simulink model "racecar_shiftlight"  (R2023b)
settings: Solver=FixedStepAuto  StartTime=0.0  StopTime=1000  FixedStep=0.001  RelTol=1e-3  EnableMultiTasking=on
PreLoadFcn:
  | colow_ws2812
values from neighbouring files (symbols this model uses):
  all_blue = [blue blue blue blue blue blue blue blue blue blue blue blue blue blue zeros]    [colow_ws2812.m]
  all_green = [green green green green green green green green green green green green green green zeros]    [colow_ws2812.m]
  all_off = [one_off one_off one_off one_off one_off one_off one_off one_off one_off one_off one_off one_off one_off one_off zeros]    [colow_ws2812.m]
  all_red = [red red red red red red red red red red red red red red zeros]    [colow_ws2812.m]
  final_drive_ratio = 4.765    [colow_ws2812.m]
  red_day_all = [red_day red_day red_day red_day red_day red_day red_day red_day red_day red_day red_day red_day red_day red_day zeros]    [colow_ws2812.m]
  stage1_day = [green_day linspace(20,20,288) green_day zeros]    [colow_ws2812.m]
  stage2_day = [green_day green_day linspace(20,20,240) green_day green_day zeros]    [colow_ws2812.m]
  stage3_day = [green_day green_day red_day linspace(20,20,192) red_day green_day green_day zeros]    [colow_ws2812.m]
  stage4_day = [green_day green_day red_day red_day linspace(20,20,144) red_day red_day green_day green_day zeros]    [colow_ws2812.m]
  stage5_day = [green_day green_day red_day red_day blue_day linspace(20,20,96) blue_day red_day red_day green_day green_day zeros]    [colow_ws2812.m]
  stage6_day = [green_day green_day red_day red_day blue_day blue_day linspace(20,20,48) blue_day blue_day red_day red_day green_day green_day zeros]    [colow_ws2812.m]
  stage7_day = [green_day green_day red_day red_day blue_day blue_day blue_day blue_day blue_day blue_day red_day red_day green_day green_day zeros]    [colow_ws2812.m]
  tire_radius = 0.31265    [colow_ws2812.m]
undefined symbols (not defined in the file or in its folder): Down, epwmFrequency, GPTRIP1SEL, GPTRIP2SEL, TZ1, TZ2, Up
libraries: simulink x12, c280xlib x6, canmsglib x6, c2837xDlib x2, c2802xlib x1
settings Model: ExtModeTrigDuration=8  Creator=LinF  LastModifiedBy=LinF
settings OptimizationCC: DefaultUnderspecifiedDataType=single  EnhancedBackFolding=on  PassReuseOutputArgsAs=Individual arguments  MaxStackSize=1024  OptimizeBlockOrder=speed  DifferentSizesBufferReuse=on  OptimizationCustomize=off  EfficientTunableParamExpr=on
settings DebuggingCC: ParameterTunabilityLossMsg=error
settings HardwareCC: ProdBitPerChar=16  ProdBitPerInt=16  ProdBitPerPointer=32  ProdBitPerSizeT=32  ProdBitPerPtrDiffT=32  ProdLargestAtomicInteger=Integer  ProdLargestAtomicFloat=None  ProdWordSize=16  ProdLongLongMode=on  ProdHWDeviceType=Texas Instruments->C2000  HardwareBoardFeatureSet=SoCBlockset
settings ModelReferenceCC: ModelReferenceNumInstancesAllowed=Single
settings SFSimCC: MATLABDynamicMemAlloc=off
settings RTWCC: Description=Embedded Coder  SystemTargetFile=ert.tlc  HardwareBoard=TI Delfino F28379D LaunchPad  TemplateMakefile=ert_default_tmf  Toolchain=Texas Instruments Code Composer Studio (C2000)  CodeProfilingSaveOptions=MetricsOnly
settings CodeAppCC: ForceParamTrailComments=on  IgnoreCustomStorageClasses=off  OperatorAnnotations=on  SimulinkDataObjDesc=on  SFDataObjDesc=on  InsertBlockDesc=on
settings ERTTargetCC: CodeReplacementLibrary=TI C28x  ExtModeTransport=4  ExtModeStaticAlloc=on  ExtModeAutomaticAllocSize=off  ExtModeStaticAllocSize=10000  ExtModeMexFile=ext_xcp  ExtModeIntrfLevel=Level2 - Open

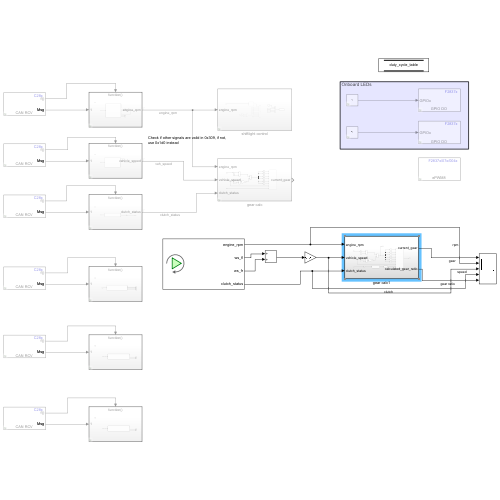
[thumbnail: Simulink's stored preview of the top-level diagram]
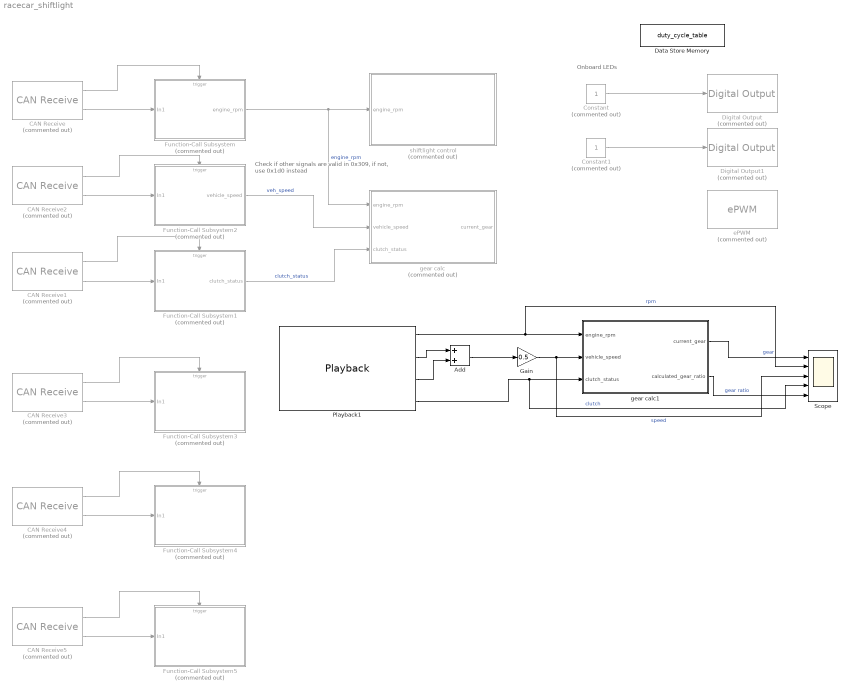
== system racecar_shiftlight ==
  note: Check if other signals are valid in 0x309, if not,
      | use 0x1d0 instead
  note: Onboard LEDs
  Add : Sum
  CAN Receive : c280xlib/CAN Receive  Commented=on  chipFamily=C280x  useModule=CAN_B  mailboxNo=0  messageID=hex2dec('17c')  messageType=Standard (11-bit identifier)  enableAcceptanceFiltering=off  messageIDMask=0  sampleTime=-1  dataType=CAN_MESSAGE_TYPE  outputAction=Output last received values  initValue=0  outputMessageID=off  outputMessageLength=off  outputMessageTimeStamp=off  postInterrupt=off  interruptLine=0
      settings: LibrarySourceBlock=c2837xDlib/CAN Receive
  CAN Receive1 : c280xlib/CAN Receive  Commented=on  chipFamily=C280x  useModule=CAN_B  mailboxNo=2  messageID=hex2dec('13c')  messageType=Standard (11-bit identifier)  enableAcceptanceFiltering=off  messageIDMask=0  sampleTime=-1  dataType=CAN_MESSAGE_TYPE  outputAction=Output last received values  initValue=0  outputMessageID=off  outputMessageLength=off  outputMessageTimeStamp=off  postInterrupt=off  interruptLine=0
      settings: LibrarySourceBlock=c2837xDlib/CAN Receive
  CAN Receive2 : c280xlib/CAN Receive  Commented=on  chipFamily=C280x  useModule=CAN_B  mailboxNo=1  messageID=hex2dec('309')  messageType=Standard (11-bit identifier)  enableAcceptanceFiltering=off  messageIDMask=0  sampleTime=-1  dataType=CAN_MESSAGE_TYPE  outputAction=Output last received values  initValue=0  outputMessageID=off  outputMessageLength=off  outputMessageTimeStamp=off  postInterrupt=off  interruptLine=0
      settings: LibrarySourceBlock=c2837xDlib/CAN Receive
  CAN Receive3 : c280xlib/CAN Receive  Commented=on  chipFamily=C280x  useModule=CAN_B  mailboxNo=3  messageID=hex2dec('1d0')  messageType=Standard (11-bit identifier)  enableAcceptanceFiltering=off  messageIDMask=0  sampleTime=-1  dataType=CAN_MESSAGE_TYPE  outputAction=Output last received values  initValue=0  outputMessageID=off  outputMessageLength=off  outputMessageTimeStamp=off  postInterrupt=off  interruptLine=0
      settings: LibrarySourceBlock=c2837xDlib/CAN Receive
  CAN Receive4 : c280xlib/CAN Receive  Commented=on  chipFamily=C280x  useModule=CAN_B  mailboxNo=4  messageID=hex2dec('1ea')  messageType=Standard (11-bit identifier)  enableAcceptanceFiltering=off  messageIDMask=0  sampleTime=-1  dataType=CAN_MESSAGE_TYPE  outputAction=Output last received values  initValue=0  outputMessageID=off  outputMessageLength=off  outputMessageTimeStamp=off  postInterrupt=off  interruptLine=0
      settings: LibrarySourceBlock=c2837xDlib/CAN Receive
  CAN Receive5 : c280xlib/CAN Receive  Commented=on  chipFamily=C280x  useModule=CAN_B  mailboxNo=5  messageID=hex2dec('156')  messageType=Standard (11-bit identifier)  enableAcceptanceFiltering=off  messageIDMask=0  sampleTime=-1  dataType=CAN_MESSAGE_TYPE  outputAction=Output last received values  initValue=0  outputMessageID=off  outputMessageLength=off  outputMessageTimeStamp=off  postInterrupt=off  interruptLine=0
      settings: LibrarySourceBlock=c2837xDlib/CAN Receive
  Constant : Constant  Commented=on
  Constant1 : Constant  Commented=on
  Data Store Memory : DataStoreMemory  DataStoreName=duty_cycle_table  WriteAfterWriteMsg=warning  InitialValue=all_off  ShowAdditionalParam=off  OutDataTypeStr=uint16  Dimensions=396
  Digital Output : c2837xDlib/Digital Output  Commented=on  GPIO_Number=GPIO24~GPIO31  GPIO_Bit0=off  GPIO_BIT0_Toggle=off  GPIO_Bit1=off  GPIO_BIT1_Toggle=off  GPIO_Bit2=off  GPIO_BIT2_Toggle=off  GPIO_Bit3=off  GPIO_BIT3_Toggle=off  GPIO_Bit4=off  GPIO_BIT4_Toggle=off  GPIO_Bit5=off  GPIO_BIT5_Toggle=off  GPIO_Bit6=off  GPIO_BIT6_Toggle=off  GPIO_Bit7=on  GPIO_BIT7_Toggle=off
  Digital Output1 : c2837xDlib/Digital Output  Commented=on  GPIO_Number=GPIO32~GPIO39  GPIO_Bit0=off  GPIO_BIT0_Toggle=off  GPIO_Bit1=off  GPIO_BIT1_Toggle=off  GPIO_Bit2=on  GPIO_BIT2_Toggle=off  GPIO_Bit3=off  GPIO_BIT3_Toggle=off  GPIO_Bit4=off  GPIO_BIT4_Toggle=off  GPIO_Bit5=off  GPIO_BIT5_Toggle=off  GPIO_Bit6=off  GPIO_BIT6_Toggle=off  GPIO_Bit7=off  GPIO_BIT7_Toggle=off
  Function-Call Subsystem : Subsystem  Commented=on  TreatAsAtomicUnit=on
  Function-Call Subsystem1 : Subsystem  Commented=on  TreatAsAtomicUnit=on
  Function-Call Subsystem2 : Subsystem  Commented=on  TreatAsAtomicUnit=on
  Function-Call Subsystem3 : Subsystem  Commented=on  TreatAsAtomicUnit=on
  Function-Call Subsystem4 : Subsystem  Commented=on  TreatAsAtomicUnit=on
  Function-Call Subsystem5 : Subsystem  Commented=on  TreatAsAtomicUnit=on
  Gain : Gain  Gain=0.5
  Playback1 : Playback  NumPorts=4  PartName=793a99b5-5b81-49ab-9d78-3a6aebb216a4
  Scope : Scope  NumInputPorts=5
  ePWM : c2802xlib/ePWM  Commented=on  PwmType=C2000_Type4  useModule=ePWM8  ePWMxLINKTBPRD=Not Linked  periodUnits=Clock cycles  timerSource=Specify via dialog  timerPeriod_clk=63  timerPeriod_sec=1/epwmFrequency  tbshadow=Counter equals to zero  countingMode=Up-Down  phaseActiveEnable=Disable  phaseDirection=Count down after sync  phaseActive=0  synchronizationEnable=off  dcaevt1Sync=off  dcbevt1Sync=off  synchronizationOption=Disable  dcbevt1SyncOut=off  dcaevt1SyncOut=off  cmpdSyncOut=off  cmpcSyncOut=off  cmpbSyncOut=off  zeroSyncOut=off  swfSyncOut=off  perSynchronizationOption=Counter equals to period (CTR=PRD)  clockPrescale=1  HSclockPrescale=1  enswap=off  ePWMxAStatus=off  ePWMxAactionLogic1=Set  ePWMxAactionLogic2=Clear  ePWMxAactionLogic3=Clear  ePWMxAactionLogic4=Set  ePWMxAactionLogic5=Do nothing  ePWMxAactionLogic6=Do nothing  ePWMxACSFenable=off  ePWMxACSFvalue=Forcing disable  ePWMxASFreload=Zero  ePWMxBStatus=on  ePWMxBactionLogic1=Set  ePWMxBactionLogic2=Clear  ePWMxBactionLogic3=Clear  ePWMxBactionLogic4=Set  ePWMxBactionLogic5=Do nothing  ePWMxBactionLogic6=Do nothing  ePWMxBCSFenable=off  ePWMxBCSFvalue=Forcing disable  ePWMxBSFreload=Zero  ePWNxBOutWay=off  ePWMxLINKCMPA=ePWM8  CMPAUnits=Percentages  CMPASource=Specify via dialog  CMPAValue_per=50  CMPAValue_clk=32000  enCMPAshadow=Counter equals to zero (CTR=Zero)  ePWMxLINKCMPB=Not Linked  CMPBUnits=Clock cycles  CMPBSource=Specify via dialog  CMPBValue_per=50  CMPBValue_clk=32000  enCMPBshadow=Counter equals to zero (CTR=Zero)  ePWMxLINKCMPC=Not Linked  CMPCUnits=Clock cycles  CMPCSource=Specify via dialog  CMPCValue_per=50  CMPCValue_clk=32000  enCMPCshadow=Counter equals to zero (CTR=Zero)  ePWMxLINKCMPD=Not Linked  CMPDUnits=Clock cycles  CMPDSource=Specify via dialog  CMPDValue_per=50  CMPDValue_clk=32000  enCMPDshadow=Counter equals to zero (CTR=Zero)  enableDBePWMxA=off  enableDBePWMxB=off  enhalfcycle=off  DBpolarity=Active high (AH)  DBedgeDelay=Positive  DBSource_ePWMxA=ePWMxA  DBSource_ePWMxB=ePWMxA  DBPeriodUnits=Clock cycles  DBperiodSource=Specify via dialog  REDperiod=0  FEDperiod=0  REDperiod_sec=0  FEDperiod_sec=0  LoadModeDBRED=Immediate without using shadow  LoadModeDBFED=Immediate without using shadow  adcstartModuleA=on  adcrequestEventA=First event  adcstartEventA=Digital Compare Module A Event 1 start of conversion (DCAEVT1.soc)  adcstartEventA_type2=Counter equals to period (CTR=PRD)  adcstartModuleB=off  adcrequestEventB=First event  adcstartEventB=Counter equals to zero (CTR=Zero)  adcstartEventB_type2=Counter equals to zero (CTR=Zero)  intEn=off  intPrd=First event  intSel=Counter equals to zero (CTR=Zero)  intSel_type2=Counter equals to zero (CTR=Zero)  hrpe=off  enHRPWM=off  HRPWM_LoadMode=Counter equals to period (CTR=PRD)  HRPWM_CTLMode=Duty or Period control mode  HRPWM_EDGMode=Both edge  hrpeb=off  enHRPWMB=off  HRPWM_LoadModeB=Counter equals to zero (CTR=ZERO)  HRPWM_CTLModeB=Duty or Period control mode  HRPWM_EDGModeB=Both edge  enHRDBRED=off  enHRDBFED=off  enSFO=on  enautoconv=on  chopperEnable=off  chopperFrequency=1  chopperFirstwidth=1  chopperDuty=12.5%  tripZonesource=Specify via dialog  tzselOSHT1=off  tzselOSHT2=off  tzselOSHT3=off  tzselOSHDCAEV1=off  tzselOSHDCBEV1=off  tzselCBC1=off  tzselCBC2=off  tzselCBC3=off  tzselCBCDCAEV2=off  tzselCBCDCBEV2=off  tzselOSHT4=off  tzselOSHT5=off  tzselOSHT6=off  tzselCBC4=off  tzselCBC5=off  tzselCBC6=off  enTzOstIntr=off  enTzCbcIntr=off  enTzDCAEVT1Intr=off  enTzDCAEVT2Intr=off  enTzDCBEVT1Intr=off  enTzDCBEVT2Intr=off  ePWMxAforced=No action  ePWMxBforced=No action  DCAEVT1forced=No action  DCBEVT1forced=No action  DCAEVT2forced=No action  DCBEVT2forced=No action  dcah=Trip Zone 1 input (TZ1)  dcal=Trip Zone 2 input (TZ2)  dcbh=Trip Zone 1 input (TZ1)  dcbl=Trip Zone 2 input (TZ2)  dcah_type2=GPTRIP1SEL/(TZ1)  dcal_type2=GPTRIP2SEL/(TZ2)  dcbh_type2=GPTRIP1SEL/(TZ1)  dcbl_type2=GPTRIP2SEL/(TZ2)  gendcaevt1=Event disabled  gendcaevt2=Event disabled  gendcbevt1=Event disabled  gendcbevt2=Event disabled  dcaevt1src=DCAEVT1 with sync  dcaevt2src=DCAEVT2 with sync  dcbevt1src=DCBEVT1 with sync  dcbevt2src=DCBEVT2 with sync  pulsesel=Counter equals to zero (CTR=Zero)  blankinv=off  blankoffset=0  blankwidth=0  evsrcsel=Filtered version of DCAEVT1 (DCAEVT1FILT)  encape=off
  gear calc : Subsystem  Commented=on
  gear calc1 : Subsystem
  shiftlight control : Subsystem  Commented=on
  wires:
  Constant/1 -> Digital Output/1
  Constant1/1 -> Digital Output1/1
  CAN Receive/2 -> Function-Call Subsystem/1(In1)
  CAN Receive/1 -> Function-Call Subsystem/Trigger
  Function-Call Subsystem/1(engine_rpm) -> gear calc/1(engine_rpm), shiftlight control/1(engine_rpm)  "engine_rpm"
  CAN Receive1/2 -> Function-Call Subsystem1/1(In1)
  CAN Receive1/1 -> Function-Call Subsystem1/Trigger
  CAN Receive2/2 -> Function-Call Subsystem2/1(In1)
  CAN Receive2/1 -> Function-Call Subsystem2/Trigger
  Function-Call Subsystem2/1(vehicle_speed) -> gear calc/2(vehicle_speed)  "veh_speed"
  Function-Call Subsystem1/1(clutch_status) -> gear calc/3(clutch_status)  "clutch_status"
  CAN Receive3/2 -> Function-Call Subsystem3/1(In1)
  CAN Receive3/1 -> Function-Call Subsystem3/Trigger
  CAN Receive4/1 -> Function-Call Subsystem4/Trigger
  CAN Receive4/2 -> Function-Call Subsystem4/1(In1)
  CAN Receive5/2 -> Function-Call Subsystem5/1(In1)
  CAN Receive5/1 -> Function-Call Subsystem5/Trigger
  Playback1/1 -> Scope/2, gear calc1/1(engine_rpm)  "rpm"
  Playback1/2 -> Add/1
  Playback1/3 -> Add/2
  Add/1 -> Gain/1
  Gain/1 -> Scope/3, gear calc1/2(vehicle_speed)  "speed"
  Playback1/4 -> Scope/4, gear calc1/3(clutch_status)  "clutch"
  gear calc1/1(current_gear) -> Scope/1  "gear"
  gear calc1/2(calculated_gear_ratio) -> Scope/5  "gear ratio"

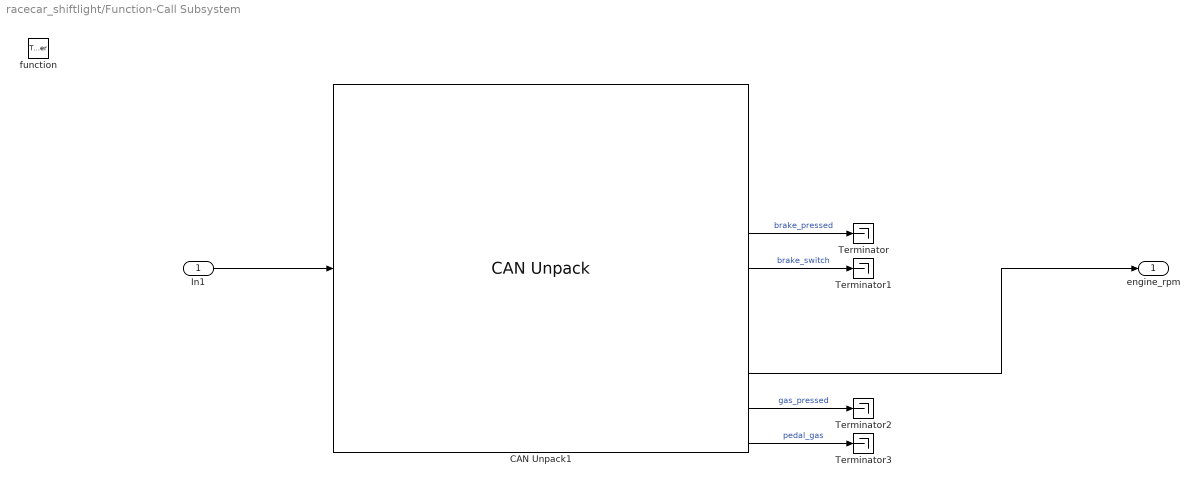
== system racecar_shiftlight/Function-Call Subsystem ==
  In1 : Inport
  function : TriggerPort  TriggerType=function-call  VariantControl=(inherit)
  CAN Unpack1 : canmsglib/CAN Unpack  CANdbFile=C:\Users\LinF\Downloads\acura_ilx_2013.dbc  MsgList=POWERTRAIN_DATA  MsgName=POWERTRAIN_DATA  MsgIDType=Standard (11-bit identifier)  MsgIdentifier=380  MsgLength=8  SignalInfo={'ACC_STATUS','38','1','BE','unsigned','Standard','0','1','0','0','1';'BOH2_17C','54','10','BE','unsigned','Standard','0','1','0','0','1';'BOH3_17C','48','5','BE','unsigned','Standard','0','1','0','0','1';'BOH_17C','33','5','BE','unsigned','Standard','0','1','0','0','1';'BRAKE_PRESSED','53','1','BE','unsigned','Standard','0','1','0','0','1';'BRAKE_SWITCH','32','1','BE','unsigned','Standard','0','1','0','0','1';'CHECKSUM','56','4','BE','unsigned','Standard','0','1','0','0','15';'COUNTER','60','2','BE','unsigned','Standard','0','1','0','0','3';'ENGINE_RPM','24','16','BE','unsigned','Standard','0','1','0','0','65535';'GAS_PRESSED','39','1','BE','unsigned','Standard','0','1','0','0','1';'PEDAL_GAS','0','8','BE','unsigned','Standard','0','1','0','0','255'}  IDPort=off  TimestampPort=off  ErrorPort=off  RemotePort=off  LengthPort=off  StatusPort=off  ApplyMinMax=off
      settings: LibrarySourceBlock=c2000lib/Target Communication/CAN Unpack  DataFormat=CANdb specified signals
  Terminator{,1..3} (4 alike) : Terminator
  engine_rpm : Outport
  wires:
  In1/1 -> CAN Unpack1/1
  CAN Unpack1/5 -> Terminator/1  "brake_pressed"
  CAN Unpack1/6 -> Terminator1/1  "brake_switch"
  CAN Unpack1/9 -> engine_rpm/1
  CAN Unpack1/10 -> Terminator2/1  "gas_pressed"
  CAN Unpack1/11 -> Terminator3/1  "pedal_gas"

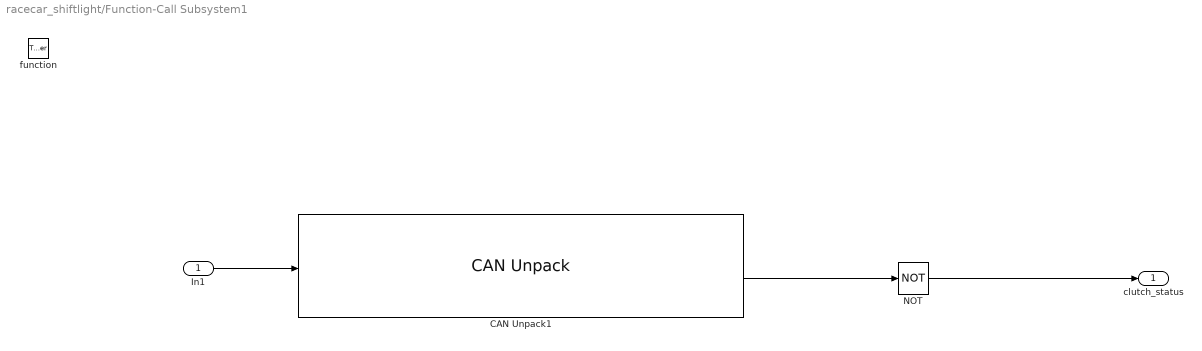
== system racecar_shiftlight/Function-Call Subsystem1 ==
  In1 : Inport
  function : TriggerPort  TriggerType=function-call  VariantControl=(inherit)
  CAN Unpack1 : canmsglib/CAN Unpack  CANdbFile=C:\Users\LinF\Downloads\acura_ilx_2013.dbc  MsgList=GAS_PEDAL  MsgName=GAS_PEDAL  MsgIDType=Standard (11-bit identifier)  MsgIdentifier=316  MsgLength=8  SignalInfo={ 'CAR_GAS', '32', '8', 'BE', 'unsigned', 'Standard', '0', '1', '0', '0', '255'; 'CHECKSUM', '56', '4', 'BE', 'unsigned', 'Standard', '0', '1', '0', '0', '15'; 'CLUTCH_STATUS_n', '50', '1', 'BE', 'unsigned', 'Standard', '0', '1', '0', '0', '1'; 'COUNTER', '60', '2', 'BE', 'unsigned', 'Standard', '0', '1', '0', '0', '3' }  IDPort=off  TimestampPort=off  ErrorPort=off  RemotePort=off  LengthPort=off  StatusPort=off  ApplyMinMax=off
      settings: LibrarySourceBlock=c2000lib/Target Communication/CAN Unpack  DataFormat=CANdb specified signals
  NOT : Logic  Operator=NOT  IconShape=distinctive  AllPortsSameDT=off  OutDataTypeStr=boolean
  clutch_status : Outport
  wires:
  In1/1 -> CAN Unpack1/1
  CAN Unpack1/3 -> NOT/1
  NOT/1 -> clutch_status/1

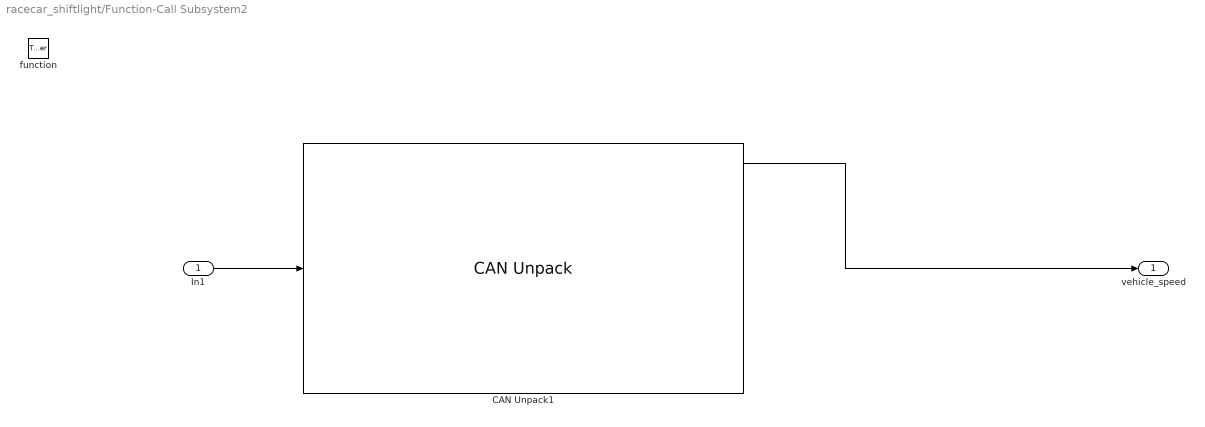
== system racecar_shiftlight/Function-Call Subsystem2 ==
  In1 : Inport
  function : TriggerPort  TriggerType=function-call  VariantControl=(inherit)
  CAN Unpack1 : canmsglib/CAN Unpack  CANdbFile=C:\Users\LinF\Downloads\acura_ilx_2013.dbc  MsgList=CAR_SPEED  MsgName=CAR_SPEED  MsgIDType=Standard (11-bit identifier)  MsgIdentifier=777  MsgLength=8  SignalInfo={'CAR_SPEED','8','16','BE','unsigned','Standard','0','0.01','0','0','65535';'CHECKSUM','56','4','BE','unsigned','Standard','0','1','0','0','15';'COUNTER','60','2','BE','unsigned','Standard','0','1','0','0','3';'IMPERIAL_UNIT','63','1','BE','unsigned','Standard','0','1','0','0','1';'LOCK_STATUS','54','2','BE','unsigned','Standard','0','1','0','0','255';'ROUGH_CAR_SPEED','16','8','BE','unsigned','Standard','0','1','0','0','255';'ROUGH_CAR_SPEED_2','24','8','BE','unsigned','Standard','0','1','0','0','255';'ROUGH_CAR_SPEED_3','40','16','BE','unsigned','Standard','0','0.01','0','0','65535'}  IDPort=off  TimestampPort=off  ErrorPort=off  RemotePort=off  LengthPort=off  StatusPort=off  ApplyMinMax=off
      settings: LibrarySourceBlock=c2000lib/Target Communication/CAN Unpack  DataFormat=CANdb specified signals
  vehicle_speed : Outport
  wires:
  In1/1 -> CAN Unpack1/1
  CAN Unpack1/1 -> vehicle_speed/1

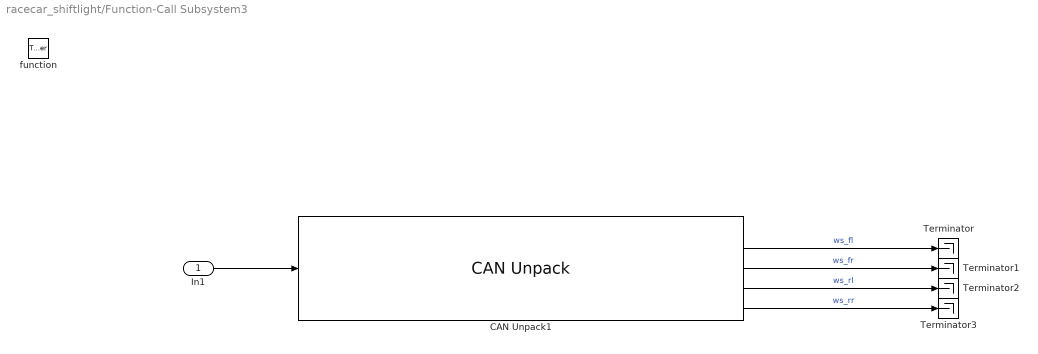
== system racecar_shiftlight/Function-Call Subsystem3 ==
  In1 : Inport
  function : TriggerPort  TriggerType=function-call  VariantControl=(inherit)
  CAN Unpack1 : canmsglib/CAN Unpack  CANdbFile=C:\Users\LinF\Downloads\acura_ilx_2013.dbc  MsgList=WHEEL_SPEEDS  MsgName=WHEEL_SPEEDS  MsgIDType=Standard (11-bit identifier)  MsgIdentifier=464  MsgLength=8  SignalInfo={'CHECKSUM','56','4','BE','unsigned','Standard','0','1','0','0','3';'WHEEL_SPEED_FL','9','15','BE','unsigned','Standard','0','0.01','0','0','250';'WHEEL_SPEED_FR','26','15','BE','unsigned','Standard','0','0.01','0','0','250';'WHEEL_SPEED_RL','43','15','BE','unsigned','Standard','0','0.01','0','0','250';'WHEEL_SPEED_RR','60','15','BE','unsigned','Standard','0','0.01','0','0','250'}  IDPort=off  TimestampPort=off  ErrorPort=off  RemotePort=off  LengthPort=off  StatusPort=off  ApplyMinMax=off
      settings: LibrarySourceBlock=c2000lib/Target Communication/CAN Unpack  DataFormat=CANdb specified signals
  Terminator{,1..3} (4 alike) : Terminator
  wires:
  In1/1 -> CAN Unpack1/1
  CAN Unpack1/2 -> Terminator/1  "ws_fl"
  CAN Unpack1/3 -> Terminator1/1  "ws_fr"
  CAN Unpack1/4 -> Terminator2/1  "ws_rl"
  CAN Unpack1/5 -> Terminator3/1  "ws_rr"

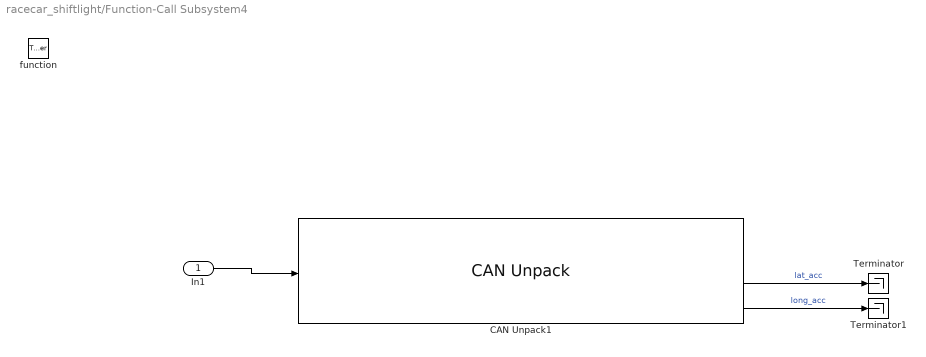
== system racecar_shiftlight/Function-Call Subsystem4 ==
  In1 : Inport
  function : TriggerPort  TriggerType=function-call  VariantControl=(inherit)
  CAN Unpack1 : canmsglib/CAN Unpack  CANdbFile=C:\Users\LinF\Downloads\acura_ilx_2013.dbc  MsgList=VEHICLE_DYNAMICS  MsgName=VEHICLE_DYNAMICS  MsgIDType=Standard (11-bit identifier)  MsgIdentifier=490  MsgLength=8  SignalInfo={'CHECKSUM','56','4','BE','unsigned','Standard','0','1','0','0','3';'COUNTER','60','2','BE','unsigned','Standard','0','1','0','0','3';'LAT_ACCEL','8','16','BE','signed','Standard','0','0.0015','0','-20','20';'LONG_ACCEL','24','16','BE','signed','Standard','0','0.0015','0','-20','20'}  IDPort=off  TimestampPort=off  ErrorPort=off  RemotePort=off  LengthPort=off  StatusPort=off  ApplyMinMax=off
      settings: LibrarySourceBlock=c2000lib/Target Communication/CAN Unpack  DataFormat=CANdb specified signals
  Terminator : Terminator
  Terminator1 : Terminator
  wires:
  In1/1 -> CAN Unpack1/1
  CAN Unpack1/3 -> Terminator/1  "lat_acc"
  CAN Unpack1/4 -> Terminator1/1  "long_acc"

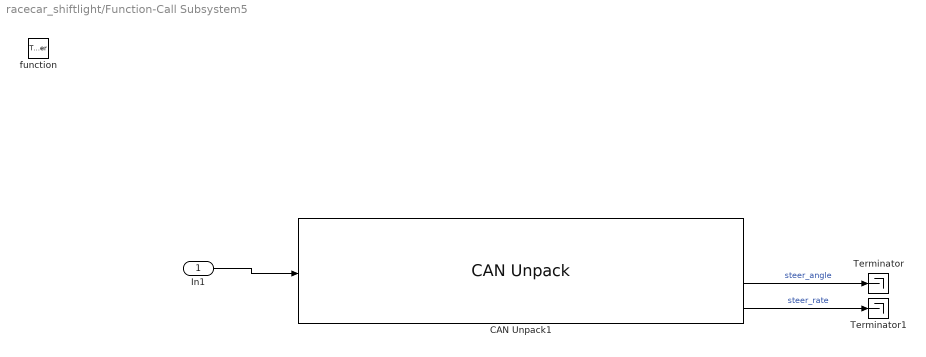
== system racecar_shiftlight/Function-Call Subsystem5 ==
  In1 : Inport
  function : TriggerPort  TriggerType=function-call  VariantControl=(inherit)
  CAN Unpack1 : canmsglib/CAN Unpack  CANdbFile=C:\Users\LinF\Downloads\acura_ilx_2013.dbc  MsgList=STEERING_SENSORS  MsgName=STEERING_SENSORS  MsgIDType=Standard (11-bit identifier)  MsgIdentifier=342  MsgLength=6  SignalInfo={'CHECKSUM','40','4','BE','unsigned','Standard','0','1','0','0','15';'COUNTER','44','2','BE','unsigned','Standard','0','1','0','0','3';'STEER_ANGLE','8','16','BE','signed','Standard','0','-0.1','0','-500','500';'STEER_ANGLE_RATE','24','16','BE','signed','Standard','0','-1','0','-3000','3000'}  IDPort=off  TimestampPort=off  ErrorPort=off  RemotePort=off  LengthPort=off  StatusPort=off  ApplyMinMax=off
      settings: LibrarySourceBlock=c2000lib/Target Communication/CAN Unpack  DataFormat=CANdb specified signals
  Terminator : Terminator
  Terminator1 : Terminator
  wires:
  In1/1 -> CAN Unpack1/1
  CAN Unpack1/3 -> Terminator/1  "steer_angle"
  CAN Unpack1/4 -> Terminator1/1  "steer_rate"

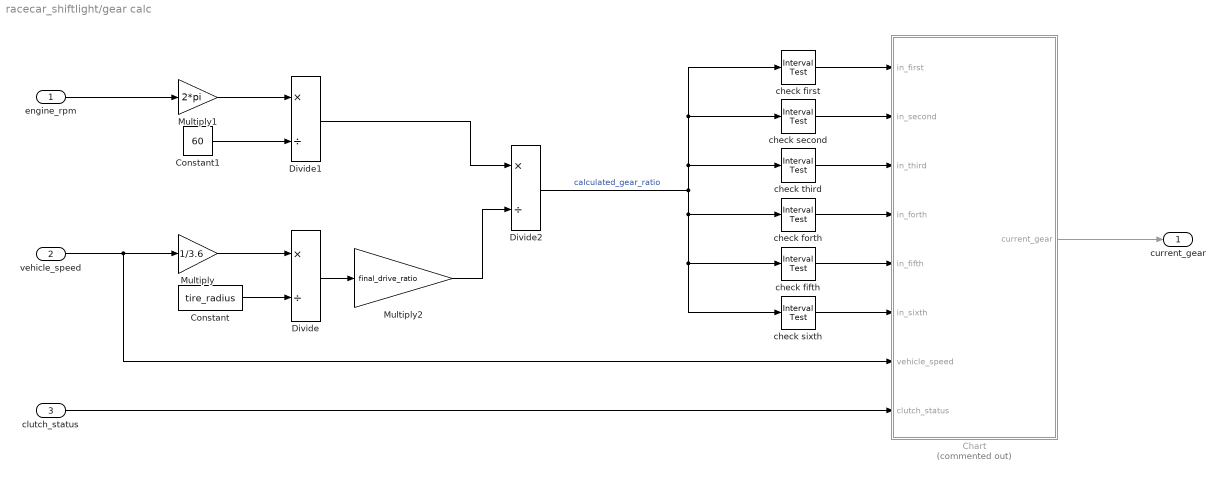
== system racecar_shiftlight/gear calc ==
  engine_rpm : Inport
  vehicle_speed : Inport  Port=2
  clutch_status : Inport  Port=3
  Chart : Stateflow chart  Commented=on  TreatAsAtomicUnit=on
      settings: PortSchema="{\"entries\":[{\"content\":{\"sides\":[{\"content\":{\"connectorIds\":[\"In2\",\"In1\",\"In3\",\"In4\",\"In5\",\"In6\",\"In7\",\"In8\"]},\"type\":\"ConnectorPlacement.EquallySpacedRectSide\",\"uuid\":\"7c5ecf18-4ca5-48cf-b6cc-f6d674adc791\"},{\"content\":{\"connectorIds\":[\"Out1\"],\"side\":\"RIGHT\"},\"type\":\"ConnectorPlacement.EquallySpacedRectSide\",\"uuid\":\"8bc4c731-54ce-4b60-a017-d200a54467ca\"},{\"content\":{\"side\":\"TOP\"},\"type\":\"ConnectorPlacement.EquallySpacedRectSide\",\"uuid\":\"b495a058-1853-40c7-b3b0-00e858c713fd\"}]},\"type\":\"ConnectorPlacement.EquallySpacedConnector\",\"uuid\":\"e858d52b-2e7f-42dc-8e65-b599dcab11be\"}],\"packageUris\":[\"http://schema.mathworks.com/mf0/Connector/R2020b\"],\"version\":\"1.0\"}"
  Constant : Constant  Value=tire_radius
  Constant1 : Constant  Value=60
  Divide : Product  Inputs=*/
  Divide1 : Product  Inputs=*/
  Divide2 : Product  Inputs=*/
  Multiply : Gain  Gain=1/3.6
  Multiply1 : Gain  Gain=2*pi
  Multiply2 : Gain  Gain=final_drive_ratio
  check fifth : simulink/Logic and Bit Operations/Interval Test  IntervalClosedRight=on  uplimit=10  IntervalClosedLeft=on  lowlimit=0  OutDataTypeStr=boolean
  check first : simulink/Logic and Bit Operations/Interval Test  IntervalClosedRight=on  uplimit=10  IntervalClosedLeft=on  lowlimit=0  OutDataTypeStr=boolean
  check forth : simulink/Logic and Bit Operations/Interval Test  IntervalClosedRight=on  uplimit=10  IntervalClosedLeft=on  lowlimit=0  OutDataTypeStr=boolean
  check second : simulink/Logic and Bit Operations/Interval Test  IntervalClosedRight=on  uplimit=10  IntervalClosedLeft=on  lowlimit=0  OutDataTypeStr=boolean
  check sixth : simulink/Logic and Bit Operations/Interval Test  IntervalClosedRight=on  uplimit=10  IntervalClosedLeft=on  lowlimit=0  OutDataTypeStr=boolean
  check third : simulink/Logic and Bit Operations/Interval Test  IntervalClosedRight=on  uplimit=10  IntervalClosedLeft=on  lowlimit=0  OutDataTypeStr=boolean
  current_gear : Outport
  wires:
  vehicle_speed/1 -> Chart/7(vehicle_speed), Multiply/1
  Multiply/1 -> Divide/1
  Constant/1 -> Divide/2
  Multiply1/1 -> Divide1/1
  Constant1/1 -> Divide1/2
  engine_rpm/1 -> Multiply1/1
  Divide1/1 -> Divide2/1
  Divide2/1 -> check third/1, check first/1, check second/1, check forth/1, check fifth/1, check sixth/1  "calculated_gear_ratio"
  Divide/1 -> Multiply2/1
  Multiply2/1 -> Divide2/2
  check first/1 -> Chart/2(in_first)
  check second/1 -> Chart/1(in_second)
  check third/1 -> Chart/3(in_third)
  check forth/1 -> Chart/4(in_forth)
  check fifth/1 -> Chart/5(in_fifth)
  check sixth/1 -> Chart/6(in_sixth)
  Chart/1(current_gear) -> current_gear/1
  clutch_status/1 -> Chart/8(clutch_status)

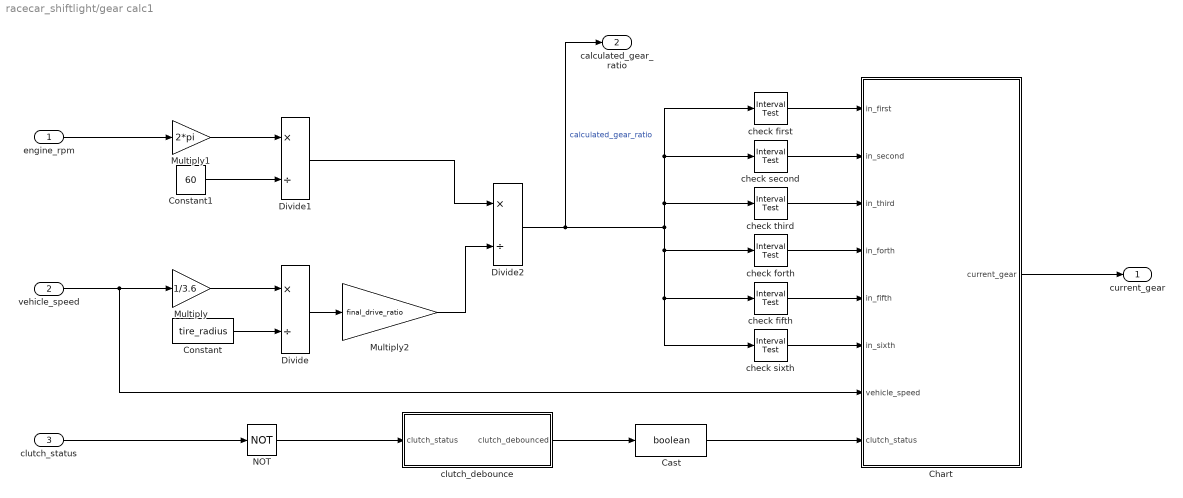
== system racecar_shiftlight/gear calc1 ==
  engine_rpm : Inport
  vehicle_speed : Inport  Port=2
  clutch_status : Inport  Port=3
  Cast : DataTypeConversion  OutDataTypeStr=boolean  SaturateOnIntegerOverflow=off  RndMeth=Floor
  Chart : Stateflow chart  TreatAsAtomicUnit=on
      settings: PortSchema="{\"entries\":[{\"content\":{\"sides\":[{\"content\":{\"connectorIds\":[\"In2\",\"In1\",\"In3\",\"In4\",\"In5\",\"In6\",\"In7\",\"In8\"]},\"type\":\"ConnectorPlacement.EquallySpacedRectSide\",\"uuid\":\"7c5ecf18-4ca5-48cf-b6cc-f6d674adc791\"},{\"content\":{\"connectorIds\":[\"Out1\"],\"side\":\"RIGHT\"},\"type\":\"ConnectorPlacement.EquallySpacedRectSide\",\"uuid\":\"8bc4c731-54ce-4b60-a017-d200a54467ca\"},{\"content\":{\"side\":\"TOP\"},\"type\":\"ConnectorPlacement.EquallySpacedRectSide\",\"uuid\":\"b495a058-1853-40c7-b3b0-00e858c713fd\"}]},\"type\":\"ConnectorPlacement.EquallySpacedConnector\",\"uuid\":\"e858d52b-2e7f-42dc-8e65-b599dcab11be\"}],\"packageUris\":[\"http://schema.mathworks.com/mf0/Connector/R2020b\"],\"version\":\"1.0\"}"
  Constant : Constant  Value=tire_radius
  Constant1 : Constant  Value=60
  Divide : Product  Inputs=*/
  Divide1 : Product  Inputs=*/
  Divide2 : Product  Inputs=*/
  Multiply : Gain  Gain=1/3.6
  Multiply1 : Gain  Gain=2*pi
  Multiply2 : Gain  Gain=final_drive_ratio
  NOT : Logic  Operator=NOT  IconShape=distinctive  AllPortsSameDT=off  OutDataTypeStr=boolean
  check fifth : simulink/Logic and Bit Operations/Interval Test  IntervalClosedRight=on  uplimit=0.88  IntervalClosedLeft=on  lowlimit=0.82  OutDataTypeStr=boolean
  check first : simulink/Logic and Bit Operations/Interval Test  IntervalClosedRight=on  uplimit=3.5  IntervalClosedLeft=on  lowlimit=3.1  OutDataTypeStr=boolean
  check forth : simulink/Logic and Bit Operations/Interval Test  IntervalClosedRight=on  uplimit=1.15  IntervalClosedLeft=on  lowlimit=1.05  OutDataTypeStr=boolean
  check second : simulink/Logic and Bit Operations/Interval Test  IntervalClosedRight=on  uplimit=2.14  IntervalClosedLeft=on  lowlimit=1.94  OutDataTypeStr=boolean
  check sixth : simulink/Logic and Bit Operations/Interval Test  IntervalClosedRight=on  uplimit=0.69  IntervalClosedLeft=on  lowlimit=0.63  OutDataTypeStr=boolean
  check third : simulink/Logic and Bit Operations/Interval Test  IntervalClosedRight=on  uplimit=1.55  IntervalClosedLeft=on  lowlimit=1.4  OutDataTypeStr=boolean
  clutch_debounce : Stateflow chart  TreatAsAtomicUnit=on
  current_gear : Outport
  calculated_gear_ratio : Outport  Port=2
  wires:
  vehicle_speed/1 -> Chart/7(vehicle_speed), Multiply/1
  Multiply/1 -> Divide/1
  Constant/1 -> Divide/2
  Multiply1/1 -> Divide1/1
  Constant1/1 -> Divide1/2
  engine_rpm/1 -> Multiply1/1
  Divide1/1 -> Divide2/1
  Divide2/1 -> calculated_gear_ratio/1, check third/1, check first/1, check second/1, check forth/1, check fifth/1, check sixth/1  "calculated_gear_ratio"
  Divide/1 -> Multiply2/1
  Multiply2/1 -> Divide2/2
  check first/1 -> Chart/2(in_first)
  check second/1 -> Chart/1(in_second)
  check third/1 -> Chart/3(in_third)
  check forth/1 -> Chart/4(in_forth)
  check fifth/1 -> Chart/5(in_fifth)
  check sixth/1 -> Chart/6(in_sixth)
  clutch_status/1 -> NOT/1
  clutch_debounce/1(clutch_debounced) -> Cast/1
  NOT/1 -> clutch_debounce/1(clutch_status)
  Chart/1(current_gear) -> current_gear/1
  Cast/1 -> Chart/8(clutch_status)

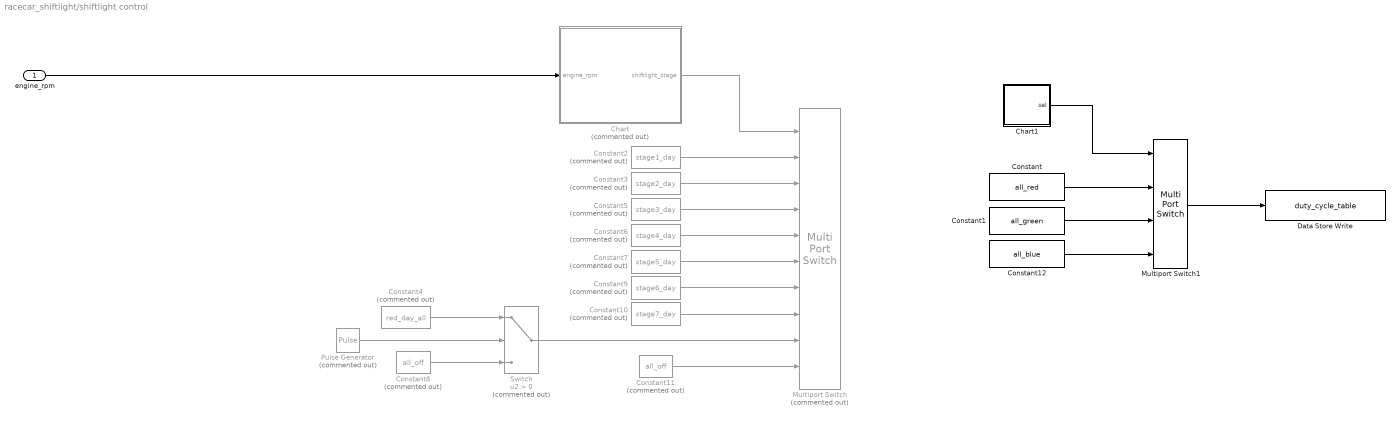
== system racecar_shiftlight/shiftlight control ==
  engine_rpm : Inport
  Chart : Stateflow chart  Commented=on  TreatAsAtomicUnit=on
  Chart1 : Stateflow chart  TreatAsAtomicUnit=on
  Constant : Constant  Value=all_red
  Constant1 : Constant  Value=all_green
  Constant10 : Constant  Commented=on  Value=stage7_day  OutDataTypeStr=uint16
  Constant11 : Constant  Commented=on  Value=all_off  OutDataTypeStr=uint16
  Constant12 : Constant  Value=all_blue
  Constant2 : Constant  Commented=on  Value=stage1_day  OutDataTypeStr=uint16
  Constant3 : Constant  Commented=on  Value=stage2_day  OutDataTypeStr=uint16
  Constant4 : Constant  Commented=on  Value=red_day_all  OutDataTypeStr=uint16
  Constant5 : Constant  Commented=on  Value=stage3_day  OutDataTypeStr=uint16
  Constant6 : Constant  Commented=on  Value=stage4_day  OutDataTypeStr=uint16
  Constant7 : Constant  Commented=on  Value=stage5_day  OutDataTypeStr=uint16
  Constant8 : Constant  Commented=on  Value=all_off  OutDataTypeStr=uint16
  Constant9 : Constant  Commented=on  Value=stage6_day  OutDataTypeStr=uint16
  Data Store Write : DataStoreWrite  DataStoreName=duty_cycle_table  IndexOptions=Index vector (dialog)  Indices=1  OutputSizes=1
  Multiport Switch : MultiPortSwitch  Commented=on  Inputs=9  DataPortIndices={5500,6000,6500,6800,0}  DiagnosticForDefault=Warning  SaturateOnIntegerOverflow=off  InputSameDT=off
  Multiport Switch1 : MultiPortSwitch  DataPortOrder=Zero-based contiguous  zeroidx=on  OutDataTypeStr=uint16  SaturateOnIntegerOverflow=off  InputSameDT=off
  Pulse Generator : DiscretePulseGenerator  Commented=on  PulseType=Time based  Period=0.15  PulseWidth=50
  Switch : Switch  Commented=on  Criteria=u2 > Threshold  SaturateOnIntegerOverflow=off  InputSameDT=off
  wires:
  Pulse Generator/1 -> Switch/2
  Constant9/1 -> Multiport Switch/7
  Constant11/1 -> Multiport Switch/10
  Constant6/1 -> Multiport Switch/5
  Chart/1(shiftlight_stage) -> Multiport Switch/1
  Constant10/1 -> Multiport Switch/8
  Constant8/1 -> Switch/3
  Switch/1 -> Multiport Switch/9
  Constant5/1 -> Multiport Switch/4
  Constant2/1 -> Multiport Switch/2
  Constant7/1 -> Multiport Switch/6
  Constant4/1 -> Switch/1
  Constant3/1 -> Multiport Switch/3
  engine_rpm/1 -> Chart/1(engine_rpm)
  Multiport Switch1/1 -> Data Store Write/1
  Chart1/1(sel) -> Multiport Switch1/1
  Constant/1 -> Multiport Switch1/2
  Constant1/1 -> Multiport Switch1/3
  Constant12/1 -> Multiport Switch1/4

== stateflow chart racecar_shiftlight/shiftlight control/Chart1 ==
  state red
    en,du:
    sel = 0;
  state green
    en,du:
    sel = 1;
  state blue
    en,du:
    sel = 2;
  (default) -> red
  red -> green : after(1,sec)
  green -> blue : after(1,sec)
  blue -> red : after(1,sec)
  data: sel output

== stateflow chart racecar_shiftlight/gear calc/Chart ==
  state Init
    en, du:
    current_gear = 0;
  state Idle
    en, du:
    current_gear = 0;
  (default) -> Init
  Idle -> Init
  Init -> Idle
  data: in_second input; in_first input; in_third input; in_forth input; in_fifth input; in_sixth input; vehicle_speed input; current_gear output; clutch_status input

== stateflow chart racecar_shiftlight/gear calc1/clutch_debounce ==
  state Wait
    state To_on
      en, du:
      clutch_debounced = 0;
    state To_off
      en, du:
      clutch_debounced = 1;
  state Off
    en, du:
    clutch_debounced = 0;
  state On
    en, du:
    clutch_debounced = 1;
  (default) -> Off
  Off -> To_on : [clutch_status == 1]
  To_on -> On [order 2] : after(100,msec)
  To_on -> Off [order 1] : [clutch_status == 0]
  To_off -> Off [order 2] : after(100,msec)
  On -> To_off : [clutch_status == 0]
  To_off -> On [order 1] : [clutch_status == 1]
  data: clutch_status input; clutch_debounced output

== stateflow chart racecar_shiftlight/shiftlight control/Chart ==
  state Init
    en, du:
    shiftlight_stage = 0;
  state stage1
    en, du:
    shiftlight_stage = 1;
  state stage2
    en, du:
    shiftlight_stage = 2;
  state stage3
    en, du:
    shiftlight_stage = 3;
  state stage4
    en, du:
    shiftlight_stage = 4;
  state stage5
    en, du:
    shiftlight_stage = 5;
  state stage6
    en, du:
    shiftlight_stage = 6;
  state stage7
    en, du:
    shiftlight_stage = 7;
  state stage8
    en, du:
    shiftlight_stage = 8;
  (default) -> Init
  Init -> stage1 : [engine_rpm >= 5400]
  stage1 -> Init [order 2] : [engine_rpm < 5400]
  stage1 -> stage2 [order 1] : [engine_rpm >= 5600]
  stage2 -> stage1 [order 1] : [engine_rpm < 5600]
  stage2 -> stage3 [order 2] : [engine_rpm >= 5800]
  stage3 -> stage2 [order 1] : [engine_rpm < 5800]
  stage3 -> stage4 [order 2] : [engine_rpm >= 6000]
  stage4 -> stage3 [order 1] : [engine_rpm < 6000]
  stage4 -> stage5 [order 2] : [engine_rpm >= 6200]
  stage5 -> stage4 [order 1] : [engine_rpm < 6200]
  stage5 -> stage6 [order 2] : [engine_rpm >= 6400]
  stage6 -> stage5 [order 1] : [engine_rpm < 6400]
  stage6 -> stage7 [order 2] : [engine_rpm >= 6600]
  stage7 -> stage6 [order 1] : [engine_rpm < 6600]
  stage7 -> stage8 [order 2] : [engine_rpm >= 6800]
  stage8 -> stage7 : [engine_rpm < 6800]
  data: engine_rpm input; shiftlight_stage output

== stateflow chart racecar_shiftlight/gear calc1/Chart ==
  state Run
    state Gear_Out
      en:
      current_gear = 0;
      du:
      if in_first
      current_gear = 1;
      elseif in_second
      current_gear = 2;
      elseif in_third
      current_gear = 3;
      elseif in_forth
      current_gear = 4;
      elseif in_fifth
      current_gear = 5;
      elseif in_sixth
      current_gear = 6;
      else
      current_gear = 0; % neutral or unknown
      end
    state Clutch_In
      en, du:
      current_gear = 0;
    state Clutch_Out
      en, du:
      current_gear = 0;
    Gear_Out -> Clutch_Out : [clutch_status == 1]
    Clutch_In -> Gear_Out : after(200,msec)
    Clutch_Out -> Clutch_In : [clutch_status == 0]
  state Init
    en, du:
    current_gear = 0;
  (default) -> Init
  Init -> Gear_Out : [vehicle_speed >= 5]
  Run -> Init : [vehicle_speed < 5]
  data: in_second input; in_first input; in_third input; in_forth input; in_fifth input; in_sixth input; vehicle_speed input; clutch_status input; current_gear output
